simulink model "Helicopter_Simulink_Model"  (R2015a)
settings: Solver=ode45  StartTime=0.0  StopTime=50  RelTol=1e-3
values from neighbouring files (symbols this model uses):
  C_0 = [[C(1,:)] ... (first row only)    [setup_lab_heli_3d_skeleton.m]
  K = lqr(A, B, Qx, Qu)    [setup_lab_heli_3d_skeleton.m]
  K_r = (-C_0*inv(A - B*K)*B)^-1    [setup_lab_heli_3d_skeleton.m]
  L_mod = place(A',C',P_L_model)'    [setup_lab_heli_3d_skeleton.m]
  Vo = -1/2*g*(-m_w*Lw + m_f*La + m_b*La ) / (La*Kf)    [setup_lab_heli_3d_skeleton.m]
undefined symbols (not defined in the file or in its folder): A, B, C, D
libraries: simulink x2
settings Model: Creator=Owner  LastModifiedBy=Owner
settings HardwareCC: TargetLongLongMode=on  TargetIntDivRoundTo=Zero  TargetEndianess=LittleEndian  TargetHWDeviceType=MATLAB Host  ProdEqTarget=off
settings RTWCC: SystemTargetFile=rsim.tlc  TemplateMakefile=rsim_default_tmf  Description=Rapid Simulation Target
settings RSimTargetCC: ERTMultiwordTypeDef=System defined  ERTMultiwordLength=256

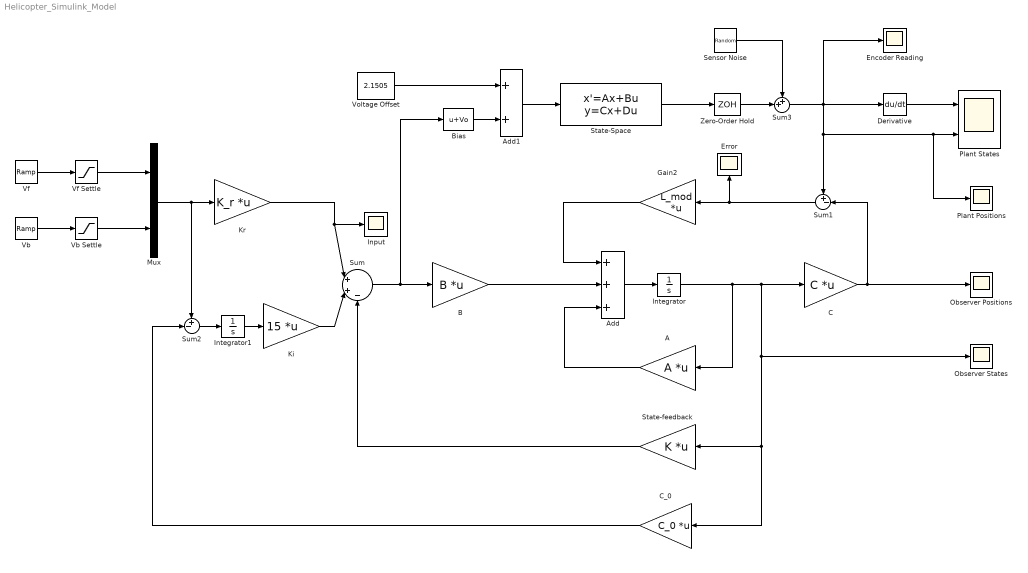
== system Helicopter_Simulink_Model ==
  A : Gain  Gain=A  Multiplication=Matrix(K*u)
  Add : Sum  Inputs=+++
  Add1 : Sum
  B : Gain  Gain=B  Multiplication=Matrix(K*u)
  Bias : Bias  Bias=Vo
  C : Gain  Gain=C  Multiplication=Matrix(K*u)
  C_0 : Gain  Gain=C_0  Multiplication=Matrix(K*u)
  Derivative : Derivative
  Encoder Reading : Scope
      settings: SaveName=ScopeData6
  Error : Scope
      settings: SaveName=ScopeData3
  Gain2 : Gain  Gain=L_mod  Multiplication=Matrix(K*u)
  Input : Scope
  Integrator : Integrator
  Integrator1 : Integrator
  Ki : Gain  Gain=15  Multiplication=Matrix(K*u)
  Kr : Gain  Gain=K_r  Multiplication=Matrix(K*u)
  Mux : Mux  Inputs=2
  Observer Positions : Scope
      settings: SaveName=ScopeData4
  Observer States : Scope
      settings: SaveName=ScopeData2
  Plant Positions : Scope
      settings: SaveName=ScopeData5
  Plant States : Scope  NumInputPorts=2
      settings: YMin=-5~-5  YMax=5~5
  Sensor Noise : UniformRandomNumber  Minimum=-0.0002  Maximum=0.0002  SampleTime=0.012
  State-Space : StateSpace  A=A  B=B  C=C  D=D  X0=0
  State-feedback : Gain  Gain=K  Multiplication=Matrix(K*u)
  Sum : Sum  Inputs=|++-
  Sum1 : Sum  Inputs=+-|
  Sum2 : Sum  Inputs=+-|
  Sum3 : Sum  Inputs=++|
  Vb : simulink/Sources/Ramp  slope=0  start=0  X0=0
  Vb Settle : Saturate  UpperLimit=0.4995  LowerLimit=-1
  Vf : simulink/Sources/Ramp  slope=0.125  start=0  X0=0
  Vf Settle : Saturate  UpperLimit=0.4995  LowerLimit=-1
  Voltage Offset : Constant  Value=2.1505
  Zero-Order Hold : ZeroOrderHold  SampleTime=0.012
  wires:
  Vf/1 -> Vf Settle/1
  Vb/1 -> Vb Settle/1
  Vf Settle/1 -> Mux/1
  Vb Settle/1 -> Mux/2
  Add1/1 -> State-Space/1
  B/1 -> Add/2
  A/1 -> Add/3
  Add/1 -> Integrator/1
  Integrator/1 -> C/1, Observer States/1, C_0/1, State-feedback/1, A/1
  Voltage Offset/1 -> Add1/1
  Bias/1 -> Add1/2
  Sum/1 -> Bias/1, B/1
  Sum3/1 -> Encoder Reading/1, Derivative/1, Sum1/1, Plant Positions/1, Plant States/2
  Gain2/1 -> Add/1
  Derivative/1 -> Plant States/1
  State-feedback/1 -> Sum/3
  C/1 -> Observer Positions/1, Sum1/2
  Mux/1 -> Kr/1, Sum2/1
  Kr/1 -> Sum/1, Input/1
  Sum2/1 -> Integrator1/1
  C_0/1 -> Sum2/2
  Ki/1 -> Sum/2
  Integrator1/1 -> Ki/1
  Sum1/1 -> Error/1, Gain2/1
  Sensor Noise/1 -> Sum3/1
  State-Space/1 -> Zero-Order Hold/1
  Zero-Order Hold/1 -> Sum3/2
